simulink model "Cv_05_Problem_5"  (R2022b)
settings: Solver=VariableStepAuto  StartTime=0.0  StopTime=100  MaxStep=0.01  MinStep=0.001  RelTol=1e-3
libraries: slpidlib x2
settings Model: Creator=honza  LastModifiedBy=honza

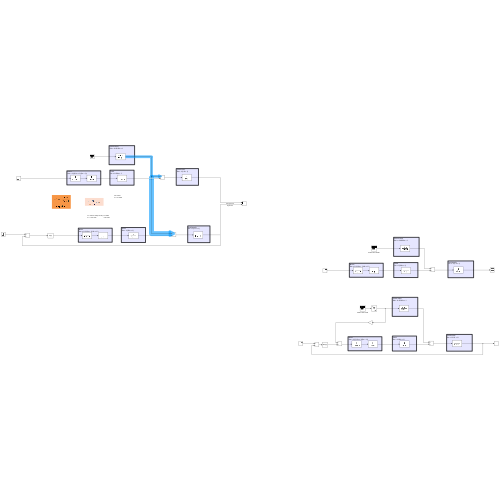
[thumbnail: Simulink's stored preview of the top-level diagram]
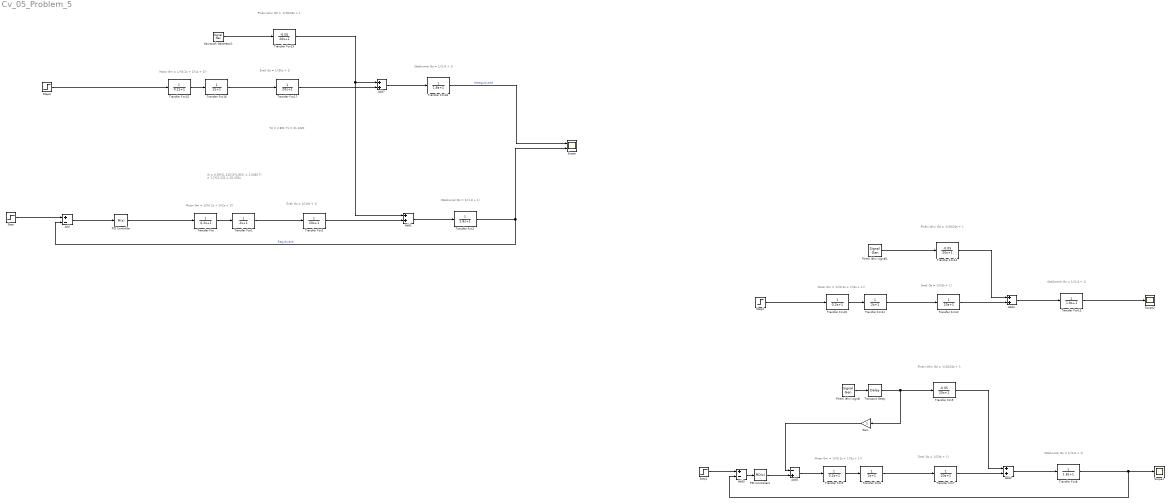
== system Cv_05_Problem_5 ==
  note: r0 = 0.35*21.232/(1*2.851)	= 2.6065
      | Ti = 1.2*21.232			= 25.4784
  note: Td = 2.851
      | T1 = 21.2320
  note: Motor
      | Gm = 1/((0.2s + 1)(2s + 1))
  note: Otáčkoměr
      | Go = 1/(1.8 + 1)
  note: Šnek
      | Gs = 1/(20s + 1)
  note: Motor
      | Gm = 1/((0.2s + 1)(2s + 1))
  note: Plnění láhví
      | Gd = -0.05/20s + 1
  note: Otáčkoměr
      | Go = 1/(1.8 + 1)
  note: Plnění láhví
      | Gd = -0.05/20s + 1
  note: Šnek
      | Gs = 1/(20s + 1)
  note: Šnek
      | Gs = 1/(20s + 1)
  note: Otáčkoměr
      | Go = 1/(1.8 + 1)
  note: Motor
      | Gm = 1/((0.2s + 1)(2s + 1))
  note: Šnek
      | Gs = 1/(20s + 1)
  note: Plnění láhví
      | Gd = -0.05/20s + 1
  note: Motor
      | Gm = 1/((0.2s + 1)(2s + 1))
  note: Otáčkoměr
      | Go = 1/(1.8 + 1)
  Add : Sum  Inputs=+-
  Add{1..2,4,7} (4 alike) : Sum
  Add3 : Sum  Inputs=+-
  Add5 : Sum  Inputs=-+
  Gain : Gain
  PID Controller : slpidlib/PID Controller  Controller=PI  Form=Ideal  TimeDomain=Continuous-time  UseExternalTs=off  SampleTime=-1  IntegratorMethod=Forward Euler  FilterMethod=Forward Euler  ControllerParametersSource=internal  P=2  I=1/20.55  UseKiTs=off  D=0  N=100  UseFilter=on  TunerSelectOption=Transfer Function Based (PID Tuner App)  InitialConditionSource=internal  InitialConditionForIntegrator=0  InitialConditionForFilter=0  DifferentiatorICPrevScaledInput=0  ExternalReset=none  TrackingMode=off  Kt=1  LimitOutput=off  SatLimitsSource=internal  UpperSaturationLimit=inf  LowerSaturationLimit=-inf  LinearizeAsGain=on  AntiWindupMode=none  Kb=1  LimitIntegrator=off  UpperIntegratorSaturationLimit=inf  LowerIntegratorSaturationLimit=-inf  POutMin=[]  POutMax=[]  IOutMin=[]  IOutMax=[]  DOutMin=[]  DOutMax=[]  NOutMin=[]  NOutMax=[]  SumOutMin=[]  SumOutMax=[]  SaturationOutMin=[]  SaturationOutMax=[]  PParamMin=[]  PParamMax=[]  IParamMin=[]  IParamMax=[]  DParamMin=[]  DParamMax=[]  NParamMin=[]  NParamMax=[]  KbParamMin=[]  KbParamMax=[]  KtParamMin=[]  KtParamMax=[]  KbOutMin=[]  KbOutMax=[]  KtOutMin=[]  KtOutMax=[]  IntegratorOutMin=[]  IntegratorOutMax=[]  FilterOutMin=[]  FilterOutMax=[]  SumI1OutMin=[]  SumI1OutMax=[]  SumI2OutMin=[]  SumI2OutMax=[]  SumI3OutMin=[]  SumI3OutMax=[]  SumI4OutMin=[]  SumI4OutMax=[]  SumDOutMin=[]  SumDOutMax=[]  DifferentiatorOutMin=[]  DifferentiatorOutMax=[]  FilterDiffOutCoefMin=[]  FilterDiffOutCoefMax=[]  ReciprocalOutMin=[]  ReciprocalOutMax=[]  SumDenOutMin=[]  SumDenOutMax=[]  SumNumOutMin=[]  SumNumOutMax=[]  DivideOutMin=[]  DivideOutMax=[]  UdiffTsProdOutMin=[]  UdiffTsProdOutMax=[]  NTsProdOutMin=[]  NTsProdOutMax=[]  UintegralTsProdOutMin=[]  UintegralTsProdOutMax=[]  UngainTsProdOutMin=[]  UngainTsProdOutMax=[]  ClampingZeroOutDataTypeStr=Inherit: Inherit via back propagation  ClampingZeroOutMin=[]  ClampingZeroOutMax=[]  FilterDenConstantOutDataTypeStr=Inherit: Inherit via back propagation  FilterDenConstantOutMin=[]  FilterDenConstantOutMax=[]  PCopyOutDataTypeStr=Inherit: Inherit via back propagation  PCopyOutMin=[]  PCopyOutMax=[]  NCopyOutDataTypeStr=Inherit: Inherit via back propagation  NCopyOutMin=[]  NCopyOutMax=[]  IntegratorContinuousStateAttributes=''  IntegratorStateMustResolveToSignalObject=off  IntegratorRTWStateStorageClass=Auto  FilterContinuousStateAttributes=''  FilterStateMustResolveToSignalObject=off  FilterRTWStateStorageClass=Auto  ParallelPVariant=Passthrough  IdealPVariant=InternalParameters  IVariant=InternalParameters  DVariant=Disabled  IntegratorVariant=Continuous  SatVariant=Disabled  AWVariant=Passthrough  PCopyVariant=Disabled  TRVariant=Disabled  FdbkBlocksVariant=Forward  IdealPFdbkVariant=Disabled  SatFdbkVariant=Disabled  DerivativeFilterVariant=Disabled  NVariant=Disabled  NCopyVariant=Disabled_SignalSpec  FilterICVariant=Disabled  IntegratorICVariant=InternalICs  ExternalResetVariant=Disabled  TRSumVariant=Passthrough  SumFdbkVariant=Disabled  SumVariant=Sum_PI  TsampFilterVariant=InternalTs  TsampNgainVariant=Passthrough  TsampIntegralVariant=Passthrough  ExternalSaturationOutDataTypeStr=Inherit: Same as second input
  PID Controller1 : slpidlib/PID Controller  Controller=PID  Form=Ideal  TimeDomain=Continuous-time  UseExternalTs=off  SampleTime=-1  IntegratorMethod=Forward Euler  FilterMethod=Forward Euler  ControllerParametersSource=internal  P=0.6*(6.028/(1*4.02))  I=1/(4*4.02)  UseKiTs=off  D=0  N=100  UseFilter=on  TunerSelectOption=Transfer Function Based (PID Tuner App)  InitialConditionSource=internal  InitialConditionForIntegrator=0  InitialConditionForFilter=0  DifferentiatorICPrevScaledInput=0  ExternalReset=none  TrackingMode=off  Kt=1  LimitOutput=off  SatLimitsSource=internal  UpperSaturationLimit=inf  LowerSaturationLimit=-inf  LinearizeAsGain=on  AntiWindupMode=none  Kb=1  LimitIntegrator=off  UpperIntegratorSaturationLimit=inf  LowerIntegratorSaturationLimit=-inf  POutMin=[]  POutMax=[]  IOutMin=[]  IOutMax=[]  DOutMin=[]  DOutMax=[]  NOutMin=[]  NOutMax=[]  SumOutMin=[]  SumOutMax=[]  SaturationOutMin=[]  SaturationOutMax=[]  PParamMin=[]  PParamMax=[]  IParamMin=[]  IParamMax=[]  DParamMin=[]  DParamMax=[]  NParamMin=[]  NParamMax=[]  KbParamMin=[]  KbParamMax=[]  KtParamMin=[]  KtParamMax=[]  KbOutMin=[]  KbOutMax=[]  KtOutMin=[]  KtOutMax=[]  IntegratorOutMin=[]  IntegratorOutMax=[]  FilterOutMin=[]  FilterOutMax=[]  SumI1OutMin=[]  SumI1OutMax=[]  SumI2OutMin=[]  SumI2OutMax=[]  SumI3OutMin=[]  SumI3OutMax=[]  SumI4OutMin=[]  SumI4OutMax=[]  SumDOutMin=[]  SumDOutMax=[]  DifferentiatorOutMin=[]  DifferentiatorOutMax=[]  FilterDiffOutCoefMin=[]  FilterDiffOutCoefMax=[]  ReciprocalOutMin=[]  ReciprocalOutMax=[]  SumDenOutMin=[]  SumDenOutMax=[]  SumNumOutMin=[]  SumNumOutMax=[]  DivideOutMin=[]  DivideOutMax=[]  UdiffTsProdOutMin=[]  UdiffTsProdOutMax=[]  NTsProdOutMin=[]  NTsProdOutMax=[]  UintegralTsProdOutMin=[]  UintegralTsProdOutMax=[]  UngainTsProdOutMin=[]  UngainTsProdOutMax=[]  ClampingZeroOutDataTypeStr=Inherit: Inherit via back propagation  ClampingZeroOutMin=[]  ClampingZeroOutMax=[]  FilterDenConstantOutDataTypeStr=Inherit: Inherit via back propagation  FilterDenConstantOutMin=[]  FilterDenConstantOutMax=[]  PCopyOutDataTypeStr=Inherit: Inherit via back propagation  PCopyOutMin=[]  PCopyOutMax=[]  NCopyOutDataTypeStr=Inherit: Inherit via back propagation  NCopyOutMin=[]  NCopyOutMax=[]  IntegratorContinuousStateAttributes=''  IntegratorStateMustResolveToSignalObject=off  IntegratorRTWStateStorageClass=Auto  FilterContinuousStateAttributes=''  FilterStateMustResolveToSignalObject=off  FilterRTWStateStorageClass=Auto  ParallelPVariant=Passthrough  IdealPVariant=InternalParameters  IVariant=InternalParameters  DVariant=InternalParameters  IntegratorVariant=Continuous  SatVariant=Disabled  AWVariant=Passthrough  PCopyVariant=Disabled  TRVariant=Disabled  FdbkBlocksVariant=Forward  IdealPFdbkVariant=Disabled  SatFdbkVariant=Disabled  DerivativeFilterVariant=ContFilter  NVariant=InternalParameters  NCopyVariant=Disabled  FilterICVariant=InternalICsFilter  IntegratorICVariant=InternalICs  ExternalResetVariant=Disabled  TRSumVariant=Passthrough  SumFdbkVariant=Disabled  SumVariant=Sum_PID  TsampFilterVariant=InternalTs  TsampNgainVariant=Passthrough  TsampIntegralVariant=Passthrough  ExternalSaturationOutDataTypeStr=Inherit: Same as second input
  Plnění láhví signál : SignalGenerator  WaveForm=sawtooth  Frequency=1/2  Units=rad/sec
  Plnění láhví signál1 : SignalGenerator  WaveForm=sawtooth  Frequency=1/2  Units=rad/sec
  Sawtooth Generator1 : SignalGenerator  WaveForm=sawtooth  Frequency=1/2  Units=rad/sec
  Scope : Scope  NumInputPorts=2
  Scope1 : Scope
  Scope2 : Scope
  Step{,1..3} (4 alike) : Step  Time=0  SampleTime=0
  Transfer Fcn{,5,10,15} (4 alike) : TransferFcn  Denominator=[0.2 1]
  Transfer Fcn{1,6,11,16} (4 alike) : TransferFcn  Denominator=[2 1]
  Transfer Fcn{2,7,12,17} (4 alike) : TransferFcn  Denominator=[20 1]
  Transfer Fcn{3,8,13,18} (4 alike) : TransferFcn  Denominator=[1.8 1]
  Transfer Fcn14 : TransferFcn  Numerator=[-0.05]  Denominator=[20 1]
  Transfer Fcn19 : TransferFcn  Numerator=[-0.05]  Denominator=[20 1]
  Transfer Fcn9 : TransferFcn  Numerator=[-0.05]  Denominator=[20 1]
  Transport Delay : TransportDelay  DelayTime=100
  wires:
  Step/1 -> Add/1
  Transfer Fcn1/1 -> Transfer Fcn2/1
  Add1/1 -> Transfer Fcn3/1
  Add/1 -> PID Controller/1
  Transfer Fcn3/1 -> Scope/2, Add/2  "Regulované"
  Transfer Fcn/1 -> Transfer Fcn1/1
  Transfer Fcn2/1 -> Add1/2
  Step2/1 -> Transfer Fcn10/1
  Gain/1 -> Add5/1
  Transfer Fcn12/1 -> Add4/2
  PID Controller1/1 -> Add5/2
  Transfer Fcn9/1 -> Add2/1
  Transfer Fcn14/1 -> Add4/1
  Transfer Fcn10/1 -> Transfer Fcn11/1
  Add5/1 -> Transfer Fcn5/1
  Add4/1 -> Transfer Fcn13/1
  Transfer Fcn13/1 -> Scope2/1
  Add2/1 -> Transfer Fcn8/1
  Transfer Fcn8/1 -> Add3/2, Scope1/1
  Transport Delay/1 -> Gain/1, Transfer Fcn9/1
  Transfer Fcn11/1 -> Transfer Fcn12/1
  Plnění láhví signál1/1 -> Transfer Fcn14/1
  Step1/1 -> Add3/1
  Transfer Fcn7/1 -> Add2/2
  Transfer Fcn6/1 -> Transfer Fcn7/1
  Transfer Fcn5/1 -> Transfer Fcn6/1
  Add3/1 -> PID Controller1/1
  Plnění láhví signál/1 -> Transport Delay/1
  Transfer Fcn18/1 -> Scope/1  "Neregulované"
  Transfer Fcn15/1 -> Transfer Fcn16/1
  Sawtooth Generator1/1 -> Transfer Fcn19/1
  Step3/1 -> Transfer Fcn15/1
  Transfer Fcn16/1 -> Transfer Fcn17/1
  Add7/1 -> Transfer Fcn18/1
  Transfer Fcn17/1 -> Add7/2
  PID Controller/1 -> Transfer Fcn/1
  Transfer Fcn19/1 -> Add1/1, Add7/1
